simulink model "lab_identyfikacja"  (R2024b)
settings: Solver=VariableStepAuto  StartTime=0.0  StopTime=20000  MaxStep=1  RelTol=1e-3
values from neighbouring files (symbols this model uses):
  czas_skok = 3000    [Identyfikacja.m]
  dPg = 1000    [Identyfikacja.m]
  K = y_delta/ dPg    [Identyfikacja.m]
  T_0 = x1 - czas_skok    (= 100)    [Identyfikacja.m]
  T_p0 = (K_p*(T_wewn0)+K_d*T_zewn0)/(K_p+K_d)    (= 15)    [Identyfikacja.m]
undefined symbols (not defined in the file or in its folder): T
settings Model: Creator=userbrigh  LastModifiedBy=userbrigh

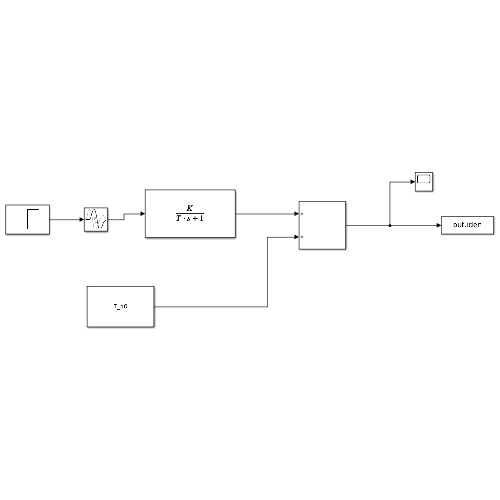
[thumbnail: Simulink's stored preview of the top-level diagram]
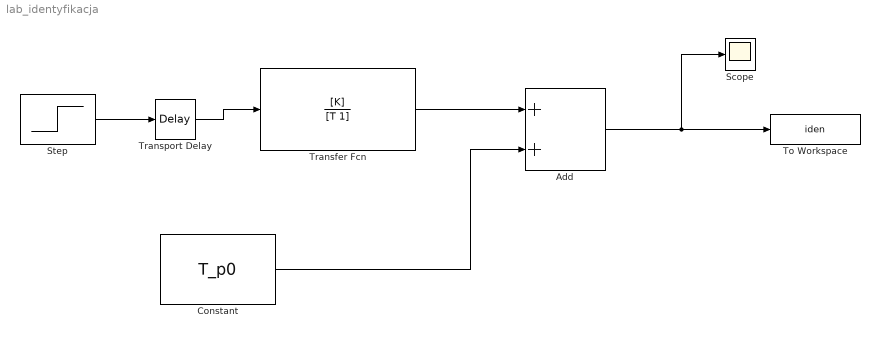
== system lab_identyfikacja ==
  Add : Sum
  Constant : Constant  Value=T_p0
  Scope : Scope
  Step : Step  Time=czas_skok  After=dPg  SampleTime=0
  To Workspace : ToWorkspace  VariableName=iden  SampleTime=-1
  Transfer Fcn : TransferFcn  Numerator=[K]  Denominator=[T 1]
  Transport Delay : TransportDelay  DelayTime=T_0
  wires:
  Constant/1 -> Add/2
  Transfer Fcn/1 -> Add/1
  Add/1 -> To Workspace/1, Scope/1
  Transport Delay/1 -> Transfer Fcn/1
  Step/1 -> Transport Delay/1
